simulink model "crazyflie Kopie"  (R2018b)
settings: Solver=FixedStepDiscrete  StartTime=0.0  StopTime=25  FixedStep=0.01  RelTol=1e-3
values from neighbouring files (symbols this model uses):
  KLQR = dlqr(sysd.A,sysd.B,Q,R)    [LQRcontrol.m]
undefined symbols (not defined in the file or in its folder): DiscIntNeverNeededParam
settings Model: PauseTimes=7  Creator=Zrean  LastModifiedBy=Jonas
settings OptimizationCC: DefaultParameterBehavior=Inlined  UseDivisionForNetSlopeComputation=on  UseFloatMulNetSlope=on  UseSpecifiedMinMax=on  InlineInvariantSignals=on  PassReuseOutputArgsAs=Individual arguments  ZeroExternalMemoryAtStartup=off  ZeroInternalMemoryAtStartup=off  NoFixptDivByZeroProtection=on  EfficientFloat2IntCast=on  LifeSpan=1
settings DebuggingCC: AlgebraicLoopMsg=error  ParameterTunabilityLossMsg=error
settings HardwareCC: ProdBitPerPointer=32  ProdBitPerSizeT=32  ProdBitPerPtrDiffT=32  ProdLargestAtomicInteger=Long  ProdLargestAtomicFloat=Double  ProdWordSize=32  ProdHWDeviceType=ARM Compatible->ARM Cortex
settings SFSimCC: SimUseLocalCustomCode=off  MATLABDynamicMemAlloc=off
settings RTWCC: SystemTargetFile=ert.tlc  GenCodeOnly=on  TemplateMakefile=ert_default_tmf  GenerateReport=on  RTWUseLocalCustomCode=off  BuildConfiguration=Faster Runs  IncludeHyperlinkInReport=on  LaunchReport=on  GenerateTraceInfo=on  GenerateTraceReport=on  GenerateTraceReportSl=on  GenerateTraceReportSf=on  GenerateTraceReportEml=on  GenerateCodeMetricsReport=on
settings CodeAppCC: ForceParamTrailComments=on  IgnoreCustomStorageClasses=off  OperatorAnnotations=on  SimulinkDataObjDesc=on  SFDataObjDesc=on  MATLABFcnDesc=on  CustomSymbolStrGlobalVar=rt$N$M  CustomSymbolStrType=$N$M  CustomSymbolStrFcn=$N$M$F  CustomSymbolStrMacro=$N$M  InsertBlockDesc=on  StateflowObjectComments=on  MATLABSourceComments=on
settings ERTTargetCC: TargetLangStandard=C99 (ISO)  MultiwordLength=2048  CombineSignalStateStructs=on  SuppressErrorStatus=on  SupportAbsoluteTime=off  SupportNonFinite=off  SupportComplex=off  InlinedParameterPlacement=NonHierarchical  ERTCustomFileTemplate=crazyflie_wrapper.tlc  ERTFilePackagingFormat=CompactWithDataFile
settings SimscapeCC: SimscapeNormalizeSystem=off

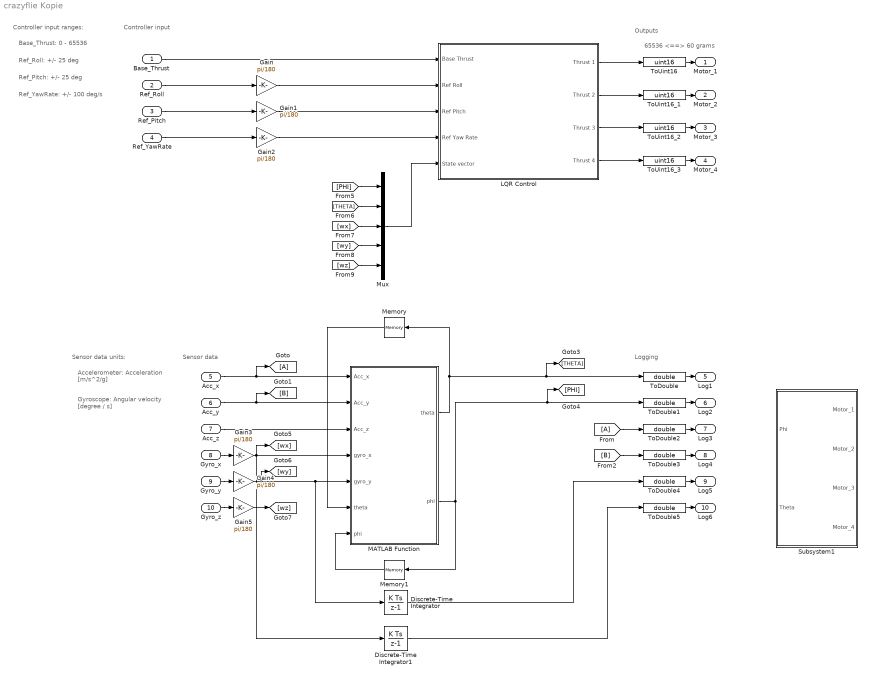
== system crazyflie Kopie ==
  note: 65536 <==> 60 grams
  note: Logging
  note: Outputs
  note: Sensor data
  note: Controller input
  note: Ref_Roll: +/- 25 deg
  note: Base_Thrust: 0 - 65536
  note: Ref_Pitch: +/- 25 deg
  note: Ref_YawRate: +/- 100 deg/s
  note: Controller input ranges:
  note: Gyroscope:
      | Angular velocity [degree / s]
  note: Accelerometer:
      | Acceleration [m/s^2/g]
  note: Sensor data units:
  Base_Thrust : Inport  OutDataTypeStr=double
  Ref_Roll : Inport  Port=2  OutDataTypeStr=double
  Ref_Pitch : Inport  Port=3  OutDataTypeStr=double
  Ref_YawRate : Inport  Port=4  OutDataTypeStr=double
  Acc_x : Inport  Port=5  OutDataTypeStr=double  PortDimensions=1
  Acc_y : Inport  Port=6  OutDataTypeStr=double  PortDimensions=1
  Acc_z : Inport  Port=7  OutDataTypeStr=double  PortDimensions=1
  Gyro_x : Inport  Port=8  OutDataTypeStr=double  PortDimensions=1
  Gyro_y : Inport  Port=9  OutDataTypeStr=double  PortDimensions=1
  Gyro_z : Inport  Port=10  OutDataTypeStr=double  PortDimensions=1
  Discrete-Time Integrator : DiscreteIntegrator  SampleTime=-1  ICPrevOutput=DiscIntNeverNeededParam  ICPrevScaledInput=DiscIntNeverNeededParam
  Discrete-Time Integrator1 : DiscreteIntegrator  SampleTime=-1  ICPrevOutput=DiscIntNeverNeededParam  ICPrevScaledInput=DiscIntNeverNeededParam
  Gain{,1..5} (6 alike) : Gain  Gain=pi/180
  LQR Control : Subsystem
  MATLAB Function : MATLAB Function  TreatAsAtomicUnit=on
  Memory : Memory
  Memory1 : Memory
  Mux : Mux  Inputs=5
  Subsystem1 : Subsystem
  ToDouble{,1..5} (6 alike) : DataTypeConversion  OutDataTypeStr=double  SaturateOnIntegerOverflow=on
  ToUint16 : DataTypeConversion  OutDataTypeStr=uint16  SaturateOnIntegerOverflow=on
  ToUint16_1 : DataTypeConversion  OutDataTypeStr=uint16  SaturateOnIntegerOverflow=on
  ToUint16_2 : DataTypeConversion  OutDataTypeStr=uint16  SaturateOnIntegerOverflow=on
  ToUint16_3 : DataTypeConversion  OutDataTypeStr=uint16  SaturateOnIntegerOverflow=on
  Motor_1 : Outport  OutDataTypeStr=uint16  LockScale=on
  Motor_2 : Outport  Port=2  OutDataTypeStr=uint16  LockScale=on
  Motor_3 : Outport  Port=3  OutDataTypeStr=uint16  LockScale=on
  Motor_4 : Outport  Port=4  OutDataTypeStr=uint16  LockScale=on
  Log1 : Outport  Port=5  OutDataTypeStr=double
  Log2 : Outport  Port=6  OutDataTypeStr=double
  Log3 : Outport  Port=7  OutDataTypeStr=double
  Log4 : Outport  Port=8  OutDataTypeStr=double
  Log5 : Outport  Port=9  OutDataTypeStr=double
  Log6 : Outport  Port=10  OutDataTypeStr=double
  wires:
  ToUint16/1 -> Motor_1/1
  ToUint16_1/1 -> Motor_2/1
  ToUint16_2/1 -> Motor_3/1
  ToUint16_3/1 -> Motor_4/1
  ToDouble/1 -> Log1/1
  ToDouble1/1 -> Log2/1
  ToDouble2/1 -> Log3/1
  ToDouble3/1 -> Log4/1
  ToDouble4/1 -> Log5/1
  ToDouble5/1 -> Log6/1
  MATLAB Function/1(theta) -> Memory/1, [THETA], ToDouble/1
  Memory1/1 -> MATLAB Function/7("phi ")
  Memory/1 -> MATLAB Function/6("theta ")
  Acc_x/1 -> [A], MATLAB Function/1(Acc_x)
  Acc_y/1 -> [B], MATLAB Function/2(Acc_y)
  Acc_z/1 -> MATLAB Function/3(Acc_z)
  Gyro_y/1 -> Gain4/1
  Discrete-Time Integrator/1 -> ToDouble4/1
  Gyro_x/1 -> Gain3/1
  Discrete-Time Integrator1/1 -> ToDouble5/1
  Base_Thrust/1 -> LQR Control/1(Base Thrust)
  LQR Control/1(Thrust 1) -> ToUint16/1
  LQR Control/2(Thrust 2) -> ToUint16_1/1
  LQR Control/3(Thrust 3) -> ToUint16_2/1
  LQR Control/4(Thrust 4) -> ToUint16_3/1
  Mux/1 -> LQR Control/5(State vector)
  [A] -> ToDouble2/1
  [B] -> ToDouble3/1
  MATLAB Function/2(phi) -> [PHI], ToDouble1/1, Memory1/1
  [PHI] -> Mux/1
  [THETA] -> Mux/2
  Gyro_z/1 -> Gain5/1
  Ref_Roll/1 -> Gain/1
  Ref_Pitch/1 -> Gain1/1
  [wx] -> Mux/3
  [wy] -> Mux/4
  [wz] -> Mux/5
  Gain/1 -> LQR Control/2(Ref Roll)
  Gain1/1 -> LQR Control/3(Ref Pitch)
  Ref_YawRate/1 -> Gain2/1
  Gain2/1 -> LQR Control/4(Ref Yaw Rate)
  Gain3/1 -> MATLAB Function/4(gyro_x), [wx], Discrete-Time Integrator1/1
  Gain4/1 -> [wy], MATLAB Function/5(gyro_y), Discrete-Time Integrator/1
  Gain5/1 -> [wz]

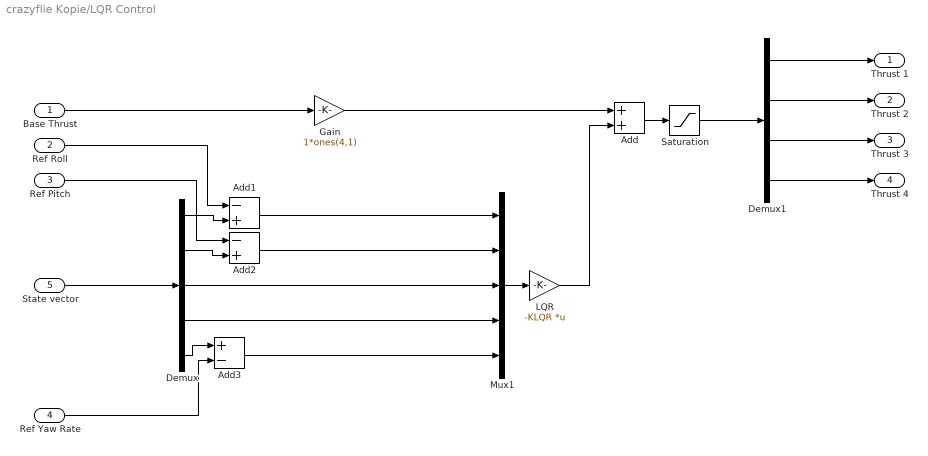
== system crazyflie Kopie/LQR Control ==
  Base Thrust : Inport
  Ref Roll : Inport  Port=2
  Ref Pitch : Inport  Port=3
  Ref Yaw Rate : Inport  Port=4
  State vector : Inport  Port=5
  Add : Sum
  Add1 : Sum  Inputs=-+
  Add2 : Sum  Inputs=-+
  Add3 : Sum  Inputs=+-
  Demux : Demux  Outputs=5
  Demux1 : Demux
  Gain : Gain  Gain=1*ones(4,1)
  LQR : Gain  Gain=-KLQR  Multiplication=Matrix(K*u)
  Mux1 : Mux  Inputs=5
  Saturation : Saturate  UpperLimit=65536  LowerLimit=0
  Thrust 1 : Outport
  Thrust 2 : Outport  Port=2
  Thrust 3 : Outport  Port=3
  Thrust 4 : Outport  Port=4
  wires:
  Demux1/4 -> Thrust 4/1
  Demux1/1 -> Thrust 1/1
  Demux1/2 -> Thrust 2/1
  Demux1/3 -> Thrust 3/1
  State vector/1 -> Demux/1
  Mux1/1 -> LQR/1
  LQR/1 -> Add/2
  Demux/3 -> Mux1/3
  Demux/4 -> Mux1/4
  Base Thrust/1 -> Gain/1
  Add/1 -> Saturation/1
  Gain/1 -> Add/1
  Saturation/1 -> Demux1/1
  Demux/1 -> Add1/2
  Ref Roll/1 -> Add1/1
  Ref Pitch/1 -> Add2/1
  Demux/2 -> Add2/2
  Add1/1 -> Mux1/1
  Add2/1 -> Mux1/2
  Demux/5 -> Add3/1
  Ref Yaw Rate/1 -> Add3/2
  Add3/1 -> Mux1/5

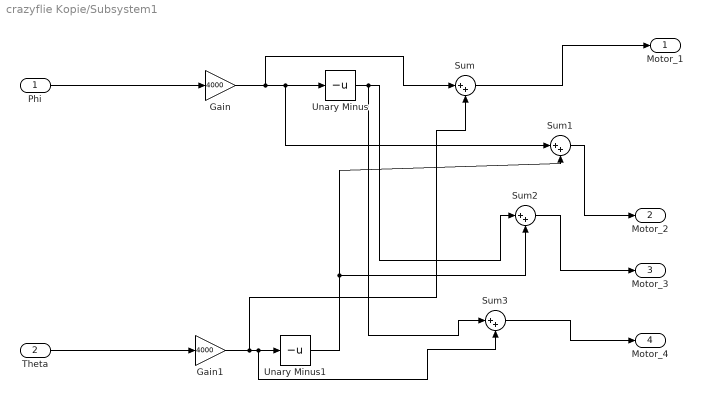
== system crazyflie Kopie/Subsystem1 ==
  Phi : Inport
  Theta : Inport  Port=2
  Gain : Gain  Gain=4000
  Gain1 : Gain  Gain=4000
  Sum{,1..3} (4 alike) : Sum  Inputs=|++
  Unary Minus : UnaryMinus
  Unary Minus1 : UnaryMinus
  Motor_1 : Outport  OutDataTypeStr=double  LockScale=on
  Motor_2 : Outport  Port=2  OutDataTypeStr=double  LockScale=on
  Motor_3 : Outport  Port=3  OutDataTypeStr=double  LockScale=on
  Motor_4 : Outport  Port=4  OutDataTypeStr=double  LockScale=on
  wires:
  Phi/1 -> Gain/1
  Theta/1 -> Gain1/1
  Gain1/1 -> Sum/2, Sum3/2, Unary Minus1/1
  Gain/1 -> Sum/1, Sum1/1, Unary Minus/1
  Sum1/1 -> Motor_2/1
  Unary Minus/1 -> Sum2/1, Sum3/1
  Unary Minus1/1 -> Sum1/2, Sum2/2
  Sum/1 -> Motor_1/1
  Sum2/1 -> Motor_3/1
  Sum3/1 -> Motor_4/1

== matlab function crazyflie Kopie/MATLAB Function ==
  data: Acc_x input; theta output; Acc_y input; Acc_z input; gyro_x input; gyro_y input; theta input; phi input; phi output
function [theta,phi] = fcn(Acc_x,Acc_y,Acc_z,gyro_x,gyro_y,theta,phi)
gamma = 0.95;
h = 0.01;

fx = Acc_x/sqrt(Acc_x^2 + Acc_y^2 + Acc_z^2);
fy = Acc_y/sqrt(Acc_x^2 + Acc_y^2 + Acc_z^2);
fz = Acc_z/sqrt(Acc_x^2 + Acc_y^2 + Acc_z^2);

theta_a = atan2(-fx,sqrt(fy^2 + fz^2));
phi_a = atan2(fy,fz);


theta = (1-gamma)*theta_a + gamma*(theta + h*gyro_y);


phi = (1-gamma)*phi_a + gamma*(phi + h*gyro_x);
